simulink model "gm_sampleModel1599_2_sub"  (R2023a)
settings: Solver=VariableStepAuto  StartTime=0.0  StopTime=10.0  RelTol=1e-3
libraries: simulink x2
settings Model: Creator=user1  LastModifiedBy=user1
settings OptimizationCC: BlockReduction=off  ConditionallyExecuteInputs=off
settings DebuggingCC: InheritedTsInSrcMsg=none

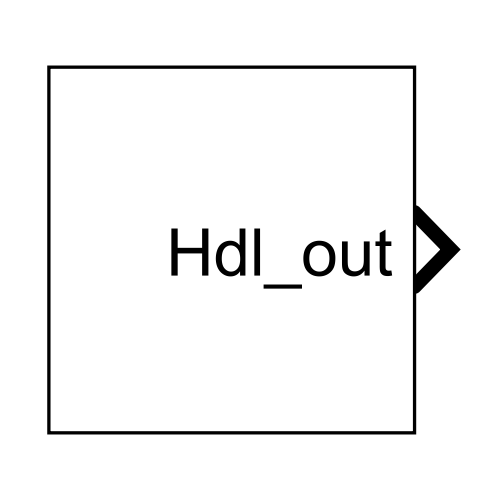
[thumbnail: Simulink's stored preview of the top-level diagram]
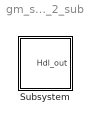
== system gm_sampleModel1599_2_sub ==
  Subsystem : Subsystem

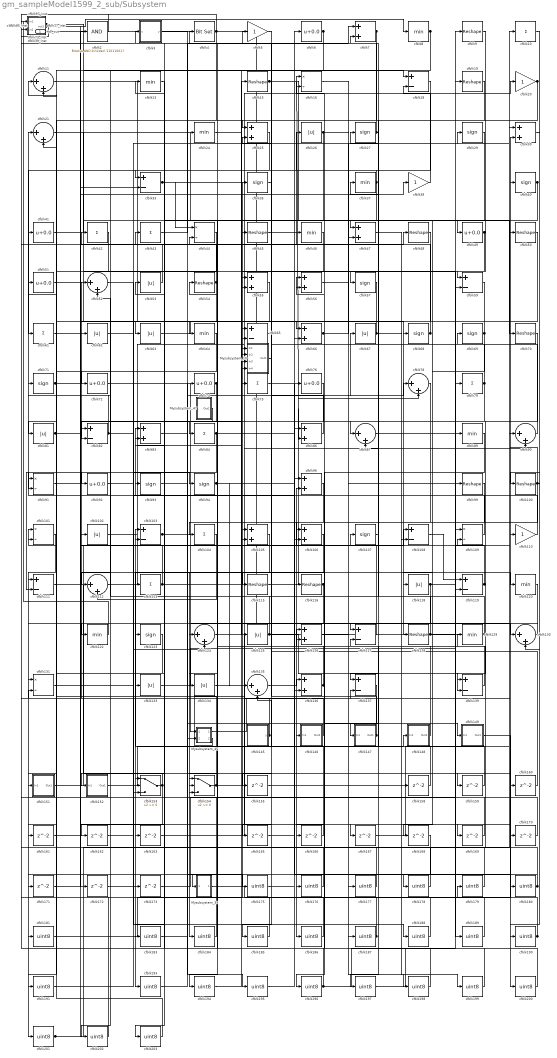
== system gm_sampleModel1599_2_sub/Subsystem ==
  Mysubsystem_10 : Subsystem
  Mysubsystem_39 : Subsystem
  Mysubsystem_45 : Subsystem
  Mysubsystem_47 : Subsystem
  cfblk1 : Constant  Value=0  OutDataTypeStr=uint8  SampleTime=1
  cfblk{10,42..43,61,75,79,84,104,113} (9 alike) : Sum  Inputs=+  OutDataTypeStr=uint8
  cfblk{9,15,19,45,48,50,54,70,99..100,115..116,128} (13 alike) : Reshape
  cfblk{16,44,91,101,109,131} (6 alike) : Product  Inputs=*/  OutDataTypeStr=uint8  RndMeth=Zero  SaturateOnIntegerOverflow=on
  cfblk{26,53,62..63,67,81,102,118,125,133..134} (11 alike) : Abs  OutDataTypeStr=uint8  SaturateOnIntegerOverflow=off
  cfblk{18,33,59,65,82,103,108,111,119,127,137,139} (12 alike) : Sum  Inputs=+-  OutDataTypeStr=uint8
  cfblk{7,25,30,47,55..56,66,83,86,96,105..106,126,136} (14 alike) : Sum  OutDataTypeStr=uint8
  cfblk{27,29,35,40,57,68..69,71,93..94,107,123} (12 alike) : Signum
  cfblk{11,21,52,78,87,90,112,124,130,135} (10 alike) : Sum  Inputs=|++  OutDataTypeStr=uint8
  cfblk{5,20,38,110} (4 alike) : Gain  OutDataTypeStr=uint8
  cfblk{8,13,24,37,46,64,89,120,122,129} (10 alike) : MinMax  OutDataTypeStr=uint8
  cfblk138_inst : Subsystem
  cfblk145 : Subsystem  mask(Counter Limited){uplimit=double(7), tsamp=double(-1)}
      mask prompts: uplimit "Simulink:masks:UpperLimit_MP"; tsamp "Simulink:masks:SampleTime_MP"
      mask help: Simulink:masks:CounterLimited_MD
      mask init:
      | nbits = double(8);
      | tsamp = double(-1);
      | uplimit = double(7);
  cfblk146 : Subsystem
  cfblk147 : Subsystem
  cfblk148 : Subsystem
  cfblk149 : Subsystem
  cfblk151 : Subsystem
  cfblk152 : Subsystem
  cfblk153 : Switch  OutDataTypeStr=uint8  SaturateOnIntegerOverflow=off  InputSameDT=off
  cfblk154 : Switch  OutDataTypeStr=uint8  SaturateOnIntegerOverflow=off  InputSameDT=off
  cfblk{155,158..163,165..173} (16 alike) : Delay  SampleTime=1
  cfblk{175..181,183..191,193..203} (27 alike) : DataTypeConversion  OutDataTypeStr=uint8  SaturateOnIntegerOverflow=off  RndMeth=Floor
  cfblk17_inst : Subsystem
  cfblk2 : simulink/Logic and Bit Operations/Bitwise Operator  logicop=AND  UseBitMask=on  BitMask=bin2dec('11011001')  BitMaskRealWorld=Stored Integer
      settings: LibrarySourceBlock=|
      | hdlsllib/Logic and Bit
      | Operations/Bitwise
      | Operator
  cfblk3 : Subsystem  mask(Compare To Zero){relop=<=, OutDataTypeStr=uint8, ZeroCross=on}
      mask prompts: relop "Simulink:masks:Operator_MP"; OutDataTypeStr "Simulink:masks:OutputDataType_MP"; ZeroCross "Simulink:masks:EnableZerocrossingDetection_MP"
      mask help: Simulink:masks:CompareToZero_MD
      mask init:
      | OutDataTypeStr = 'uint8';
      | ZeroCross = 'on';
      | blkName = 'sampleModel1599_2_sub/Subsystem/cfblk3';
      | relop = '<=';
      | setValue = 'fixdt(0, 8)';
      mask TypeOptions relop: == | ~= | < | <= | >= | >
      mask TypeOptions OutDataTypeStr: Simulink:masks:uint8 | Simulink:masks:boolean
      mask Callback ZeroCross: sl('zeroCrossEnable', gcbh);
      mask Display: disp([relop,' 0'])
  cfblk39_inst : Subsystem
  cfblk4 : simulink/Logic and Bit Operations/Bit Set  iBit=0
      settings: LibrarySourceBlock=|
      | hdlsllib/Logic and Bit
      | Operations/Bit Set
  cfblk{6,41,49,51,72,74,76,92} (8 alike) : Bias  Bias=0.0  SaturateOnIntegerOverflow=off
  cfblk73_inst : Subsystem
  cfblk77_inst : Subsystem
  cfblk85_inst : Subsystem
  cfblk97_inst : Subsystem
  Hdl_out : Outport  OutDataTypeStr=uint8  SampleTime=1
  wires:
  Mysubsystem_10/1(Out1) -> Mysubsystem_39/1(In1)
  Mysubsystem_39/1(Out1) -> cfblk30/2
  Mysubsystem_45/1(Out1) -> cfblk40/1
  Mysubsystem_45/2(Out2) -> cfblk48/1
  Mysubsystem_47/1(Out1) -> Mysubsystem_45/1(In1)
  cfblk1/1 -> cfblk87/1, cfblk63/1
  cfblk10/1 -> cfblk100/1
  cfblk100/1 -> cfblk50/1, cfblk186/1, cfblk130/2, cfblk146/1(In1)
  cfblk101/1 -> cfblk201/1
  cfblk102/1 -> cfblk20/1
  cfblk103/1 -> cfblk195/1, cfblk127/1
  cfblk104/1 -> cfblk112/2
  cfblk105/1 -> cfblk184/1
  cfblk106/1 -> cfblk193/1
  cfblk107/1 -> cfblk27/1
  cfblk108/1 -> cfblk119/1
  cfblk109/1 -> cfblk83/1
  cfblk11/1 -> cfblk128/1
  cfblk110/1 -> cfblk21/1
  cfblk111/1 -> cfblk159/1
  cfblk112/1 -> cfblk35/1
  cfblk113/1 -> cfblk52/1, cfblk15/1
  cfblk115/1 -> cfblk78/2
  cfblk116/1 -> cfblk194/1, cfblk176/1
  cfblk118/1 -> cfblk181/1, cfblk154/3, cfblk110/1
  cfblk119/1 -> cfblk52/2, cfblk109/2
  cfblk120/1 -> cfblk131/1
  cfblk122/1 -> cfblk97_inst/1(in1)
  cfblk123/1 -> cfblk151/1(In1)
  cfblk124/1 -> cfblk167/1
  cfblk125/1 -> cfblk71/1, cfblk139/2
  cfblk126/1 -> cfblk187/1
  cfblk127/1 -> cfblk96/2
  cfblk128/1 -> cfblk19/1, cfblk13/1
  cfblk129/1 -> cfblk7/2, Hdl_out/1
  cfblk13/1 -> cfblk163/1
  cfblk130/1 -> cfblk124/1
  cfblk131/1 -> cfblk173/1
  cfblk133/1 -> cfblk79/1
  cfblk134/1 -> cfblk137/2
  cfblk135/1 -> cfblk136/1
  cfblk136/1 -> cfblk85_inst/2(in2), cfblk103/1
  cfblk137/1 -> cfblk166/1
  cfblk138_inst/1(out1) -> cfblk189/1, cfblk18/1
  cfblk139/1 -> cfblk93/1
  cfblk145/1(y) -> cfblk73_inst/2(in2), cfblk62/1
  cfblk146/1(Out1) -> cfblk131/2
  cfblk147/1(Out1) -> cfblk5/1, cfblk44/2
  cfblk148/1(Out1) -> cfblk55/1
  cfblk149/1(Out1) -> cfblk200/1
  cfblk15/1 -> cfblk86/2, cfblk49/1
  cfblk151/1(Out1) -> cfblk107/1
  cfblk152/1(Out1) -> cfblk148/1(In1)
  cfblk153/1 -> cfblk162/1, cfblk152/1(In1)
  cfblk154/1 -> cfblk90/2, cfblk21/2
  cfblk155/1 -> cfblk66/2
  cfblk158/1 -> cfblk127/2
  cfblk159/1 -> cfblk103/2
  cfblk16/1 -> cfblk177/1
  cfblk160/1 -> cfblk25/2
  cfblk161/1 -> cfblk108/1
  cfblk162/1 -> cfblk188/1
  cfblk163/1 -> cfblk78/1
  cfblk165/1 -> cfblk136/2
  cfblk166/1 -> cfblk135/2
  cfblk167/1 -> cfblk90/1
  cfblk168/1 -> cfblk178/1
  cfblk169/1 -> cfblk17_inst/1(in1)
  cfblk17_inst/1(out1) -> cfblk57/1
  cfblk170/1 -> cfblk83/2
  cfblk171/1 -> cfblk59/2
  cfblk172/1 -> cfblk96/1
  cfblk173/1 -> cfblk109/1
  cfblk175/1 -> cfblk76/1
  cfblk176/1 -> cfblk3/1(u)
  cfblk177/1 -> cfblk17_inst/2(in2)
  cfblk178/1 -> cfblk16/1
  cfblk179/1 -> cfblk16/2
  cfblk18/1 -> cfblk82/2
  cfblk180/1 -> cfblk4/1, cfblk171/1, cfblk129/1
  cfblk181/1 -> cfblk75/1
  cfblk183/1 -> Mysubsystem_45/2(In2)
  cfblk184/1 -> cfblk53/1
  cfblk185/1 -> cfblk105/1
  cfblk186/1 -> cfblk105/2
  cfblk187/1 -> cfblk86/1, cfblk77_inst/2(in2)
  cfblk188/1 -> cfblk126/1
  cfblk189/1 -> cfblk126/2
  cfblk19/1 -> cfblk47/1
  cfblk190/1 -> cfblk179/1, cfblk138_inst/1(in1)
  cfblk191/1 -> cfblk30/1
  cfblk193/1 -> cfblk67/1
  cfblk194/1 -> cfblk106/1
  cfblk195/1 -> cfblk106/2
  cfblk196/1 -> cfblk97_inst/2(in2), cfblk9/1, cfblk43/1
  cfblk197/1 -> cfblk89/1
  cfblk198/1 -> cfblk54/1
  cfblk199/1 -> cfblk56/1
  cfblk2/1 -> cfblk39_inst/1(in1)
  cfblk20/1 -> cfblk81/1, cfblk203/1
  cfblk200/1 -> cfblk56/2
  cfblk201/1 -> cfblk2/1, cfblk10/1
  cfblk202/1 -> cfblk101/1
  cfblk203/1 -> cfblk101/2
  cfblk21/1 -> cfblk70/1
  cfblk24/1 -> cfblk65/1
  cfblk25/1 -> cfblk61/1
  cfblk26/1 -> cfblk99/1, cfblk165/1
  cfblk27/1 -> cfblk87/2, cfblk85_inst/1(in1), cfblk197/1
  cfblk29/1 -> cfblk147/1(In1)
  cfblk3/1(y) -> cfblk175/1
  cfblk30/1 -> cfblk190/1
  cfblk33/1 -> cfblk116/1, cfblk44/1, Mysubsystem_10/3(In3)
  cfblk35/1 -> cfblk115/1
  cfblk37/1 -> cfblk33/1, cfblk134/1
  cfblk38/1 -> cfblk18/2
  cfblk39_inst/1(out1) -> cfblk8/1
  cfblk4/1 -> cfblk73_inst/1(in1), cfblk153/1
  cfblk40/1 -> cfblk47/2, cfblk183/1
  cfblk41/1 -> cfblk24/1
  cfblk42/1 -> cfblk161/1
  cfblk43/1 -> cfblk7/1
  cfblk44/1 -> cfblk91/2
  cfblk45/1 -> cfblk26/1
  cfblk46/1 -> cfblk185/1
  cfblk47/1 -> cfblk199/1
  cfblk48/1 -> cfblk112/1
  cfblk49/1 -> cfblk55/2, Mysubsystem_10/4(In4)
  cfblk5/1 -> cfblk25/1
  cfblk50/1 -> cfblk153/3
  cfblk51/1 -> cfblk84/1
  cfblk52/1 -> cfblk124/2
  cfblk53/1 -> cfblk77_inst/1(in1)
  cfblk54/1 -> cfblk153/2, cfblk42/1
  cfblk55/1 -> cfblk91/1
  cfblk56/1 -> cfblk198/1
  cfblk57/1 -> cfblk92/1
  cfblk59/1 -> cfblk118/1
  cfblk6/1 -> Mysubsystem_10/1(In1), cfblk122/1
  cfblk61/1 -> cfblk102/1
  cfblk62/1 -> cfblk154/2
  cfblk63/1 -> cfblk66/1
  cfblk64/1 -> cfblk111/1
  cfblk65/1 -> cfblk113/1
  cfblk66/1 -> cfblk68/1, cfblk29/1, cfblk130/1
  cfblk67/1 -> cfblk72/1, cfblk169/1
  cfblk68/1 -> cfblk11/1, cfblk37/1
  cfblk69/1 -> cfblk65/2, cfblk168/1
  cfblk7/1 -> cfblk155/1, Mysubsystem_10/2(In2)
  cfblk70/1 -> cfblk139/1
  cfblk71/1 -> cfblk170/1, cfblk46/1
  cfblk72/1 -> cfblk125/1
  cfblk73_inst/1(out1) -> cfblk33/2, cfblk64/1
  cfblk74/1 -> cfblk202/1, cfblk123/1
  cfblk75/1 -> cfblk180/1
  cfblk76/1 -> cfblk133/1
  cfblk77_inst/1(out1) -> cfblk39_inst/2(in2)
  cfblk78/1 -> cfblk108/2
  cfblk79/1 -> cfblk69/1, cfblk154/1
  cfblk8/1 -> cfblk82/1, cfblk11/2
  cfblk81/1 -> cfblk191/1, cfblk119/2
  cfblk82/1 -> cfblk51/1, cfblk160/1
  cfblk83/1 -> cfblk74/1
  cfblk84/1 -> cfblk111/2, cfblk158/1
  cfblk85_inst/1(out1) -> cfblk172/1
  cfblk86/1 -> cfblk45/1
  cfblk87/1 -> cfblk120/1
  cfblk89/1 -> cfblk196/1
  cfblk9/1 -> cfblk59/1
  cfblk90/1 -> cfblk41/1
  cfblk91/1 -> cfblk38/1
  cfblk92/1 -> cfblk94/1
  cfblk93/1 -> cfblk149/1(In1)
  cfblk94/1 -> cfblk6/1, cfblk135/1
  cfblk96/1 -> cfblk104/1
  cfblk97_inst/1(out1) -> cfblk138_inst/2(in2)
  cfblk99/1 -> cfblk137/1

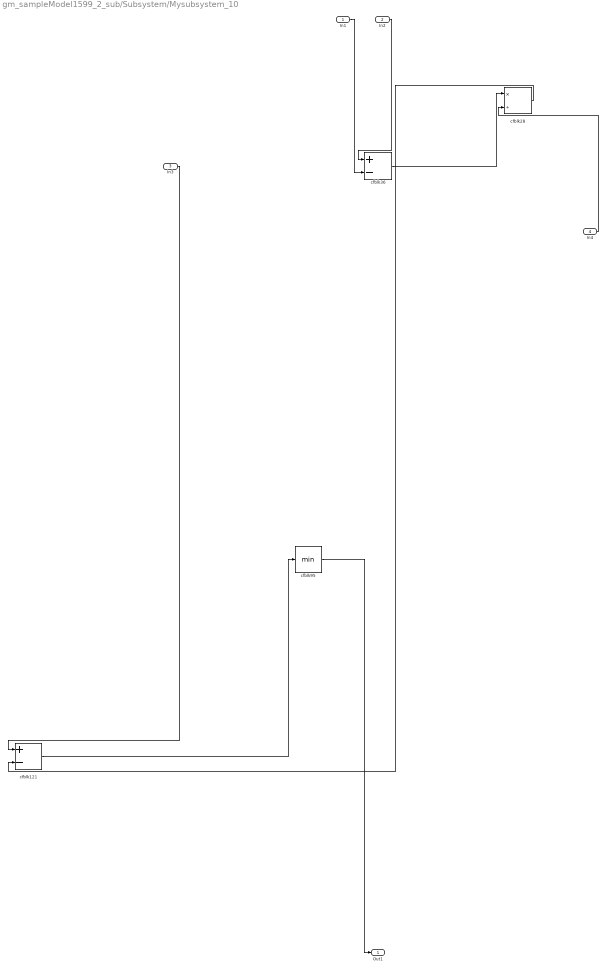
== system gm_sampleModel1599_2_sub/Subsystem/Mysubsystem_10 ==
  In1 : Inport  OutDataTypeStr=uint8  PortDimensions=1  SampleTime=1
  In2 : Inport  Port=2  OutDataTypeStr=uint8  PortDimensions=1  SampleTime=1
  In3 : Inport  Port=3  OutDataTypeStr=uint8  PortDimensions=1  SampleTime=1
  In4 : Inport  Port=4  OutDataTypeStr=uint8  PortDimensions=1  SampleTime=1
  cfblk121 : Sum  Inputs=+-
  cfblk28 : Product  Inputs=*/  RndMeth=Zero  SaturateOnIntegerOverflow=on
  cfblk36 : Sum  Inputs=+-
  cfblk95 : MinMax
  Out1 : Outport  SampleTime=1
  wires:
  In1/1 -> cfblk36/2
  In2/1 -> cfblk36/1
  In3/1 -> cfblk121/1
  In4/1 -> cfblk28/2
  cfblk121/1 -> cfblk95/1
  cfblk28/1 -> cfblk121/2
  cfblk36/1 -> cfblk28/1
  cfblk95/1 -> Out1/1

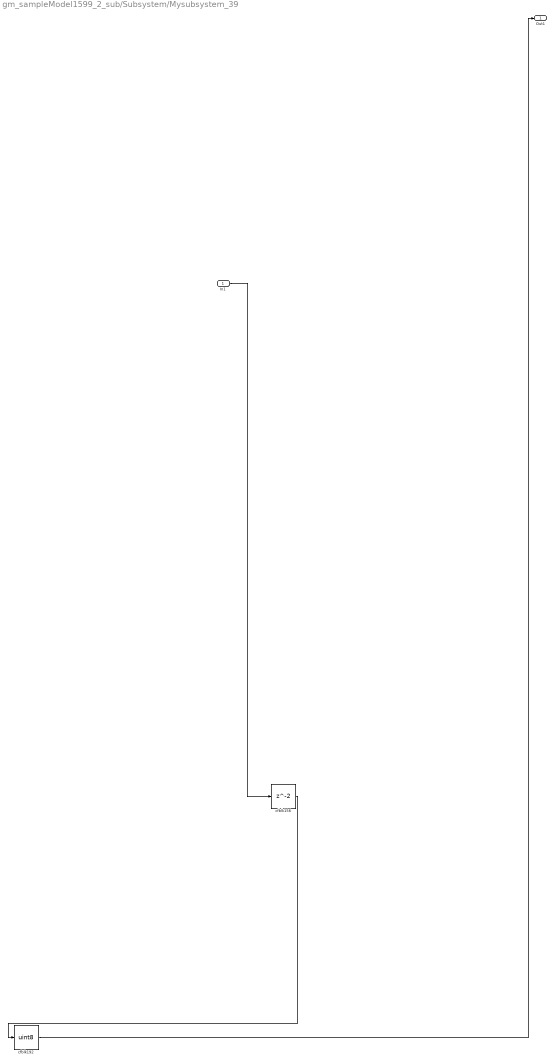
== system gm_sampleModel1599_2_sub/Subsystem/Mysubsystem_39 ==
  In1 : Inport  OutDataTypeStr=uint8  PortDimensions=1  SampleTime=1
  cfblk156 : Delay  SampleTime=1
  cfblk192 : DataTypeConversion  OutDataTypeStr=uint8  SaturateOnIntegerOverflow=off  RndMeth=Floor
  Out1 : Outport  SampleTime=1
  wires:
  In1/1 -> cfblk156/1
  cfblk156/1 -> cfblk192/1
  cfblk192/1 -> Out1/1

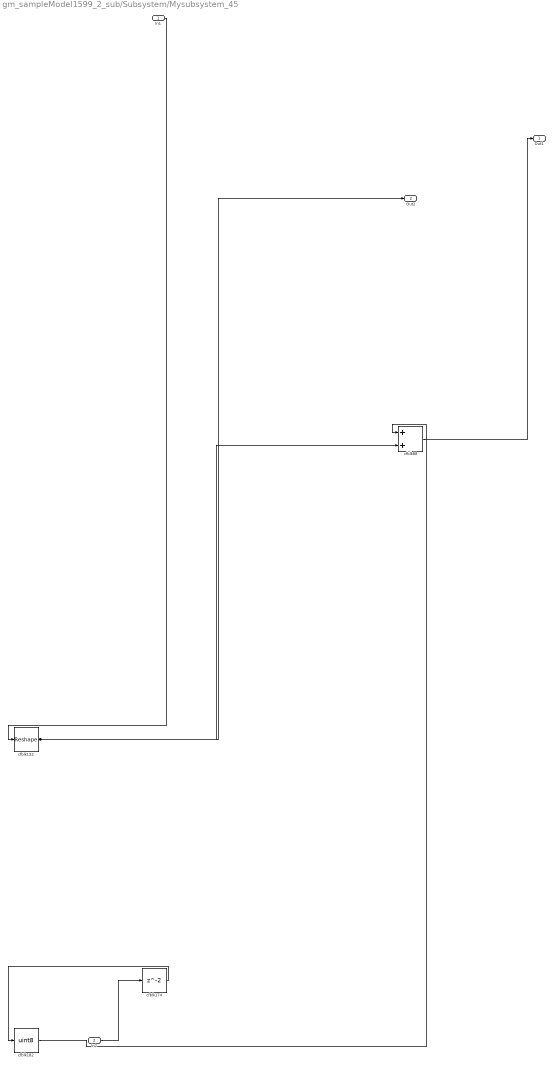
== system gm_sampleModel1599_2_sub/Subsystem/Mysubsystem_45 ==
  In1 : Inport  OutDataTypeStr=uint8  PortDimensions=1  SampleTime=1
  In2 : Inport  Port=2  OutDataTypeStr=uint8  PortDimensions=1  SampleTime=1
  cfblk132 : Reshape
  cfblk174 : Delay  SampleTime=1
  cfblk182 : DataTypeConversion  OutDataTypeStr=uint8  SaturateOnIntegerOverflow=off  RndMeth=Floor
  cfblk88 : Sum
  Out1 : Outport  SampleTime=1
  Out2 : Outport  Port=2  SampleTime=1
  wires:
  In1/1 -> cfblk132/1
  In2/1 -> cfblk174/1
  cfblk132/1 -> cfblk88/2, Out2/1
  cfblk174/1 -> cfblk182/1
  cfblk182/1 -> cfblk88/1
  cfblk88/1 -> Out1/1

== system gm_sampleModel1599_2_sub/Subsystem/Mysubsystem_47 ==
  cfblk14 : Reshape
  cfblk144 : Ground
  Out1 : Outport  SampleTime=1
  wires:
  cfblk14/1 -> Out1/1
  cfblk144/1 -> cfblk14/1

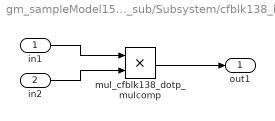
== system gm_sampleModel1599_2_sub/Subsystem/cfblk138_inst ==
  in1 : Inport  OutDataTypeStr=uint8  SampleTime=1
  in2 : Inport  Port=2  OutDataTypeStr=uint8  SampleTime=1
  mul_cfblk138_dotp_mulcomp : Product  Inputs=**  OutDataTypeStr=uint8  SampleTime=1
  out1 : Outport  OutDataTypeStr=uint8  SampleTime=1
  wires:
  in1/1 -> mul_cfblk138_dotp_mulcomp/1
  in2/1 -> mul_cfblk138_dotp_mulcomp/2
  mul_cfblk138_dotp_mulcomp/1 -> out1/1

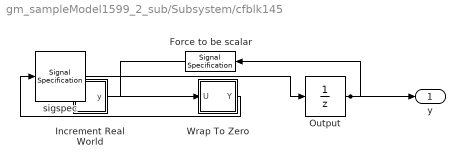
== system gm_sampleModel1599_2_sub/Subsystem/cfblk145 ==
  Force to be scalar : SignalSpecification  DisableCoverage=on  Dimensions=1
  Increment Real World : Subsystem  mask(Real World Value Increment){}
      mask help: Simulink:masks:RealWorldValueIncrement_MD
      mask Display: disp('V++')
  Output : UnitDelay  InitialCondition=0.0  SampleTime=tsamp  HasFrameUpgradeWarning=on
  Wrap To Zero : Subsystem  mask(Wrap To Zero){Threshold=double(7)}
      mask prompts: Threshold "Simulink:masks:Threshold_MP"
      mask help: Simulink:masks:WrapToZero_MD
  sigspec : SignalSpecification  OutDataTypeStr=uint8  Dimensions=1
  y : Outport  SampleTime=1
  wires:
  Force to be scalar/1 -> Increment Real World/1(u)
  Increment Real World/1(y) -> Wrap To Zero/1(U)
  Output/1 -> Force to be scalar/1, y/1
  Wrap To Zero/1(Y) -> sigspec/1
  sigspec/1 -> Output/1

== system gm_sampleModel1599_2_sub/Subsystem/cfblk146 ==
  In1 : Inport  OutDataTypeStr=uint8  PortDimensions=1  SampleTime=1
  Out1 : Outport  SampleTime=1
  wires:
  In1/1 -> Out1/1

== system gm_sampleModel1599_2_sub/Subsystem/cfblk147 ==
  In1 : Inport  OutDataTypeStr=uint8  PortDimensions=1  SampleTime=1
  Out1 : Outport  SampleTime=1
  wires:
  In1/1 -> Out1/1

== system gm_sampleModel1599_2_sub/Subsystem/cfblk148 ==
  In1 : Inport  OutDataTypeStr=uint8  PortDimensions=1  SampleTime=1
  Out1 : Outport  SampleTime=1
  wires:
  In1/1 -> Out1/1

== system gm_sampleModel1599_2_sub/Subsystem/cfblk149 ==
  In1 : Inport  OutDataTypeStr=uint8  PortDimensions=1  SampleTime=1
  Out1 : Outport  SampleTime=1
  wires:
  In1/1 -> Out1/1

== system gm_sampleModel1599_2_sub/Subsystem/cfblk151 ==
  In1 : Inport  OutDataTypeStr=uint8  PortDimensions=1  SampleTime=1
  Out1 : Outport  SampleTime=1
  wires:
  In1/1 -> Out1/1

== system gm_sampleModel1599_2_sub/Subsystem/cfblk152 ==
  In1 : Inport  OutDataTypeStr=uint8  PortDimensions=1  SampleTime=1
  Out1 : Outport  SampleTime=1
  wires:
  In1/1 -> Out1/1

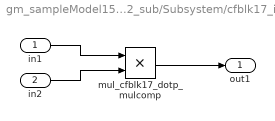
== system gm_sampleModel1599_2_sub/Subsystem/cfblk17_inst ==
  in1 : Inport  OutDataTypeStr=uint8  SampleTime=1
  in2 : Inport  Port=2  OutDataTypeStr=uint8  SampleTime=1
  mul_cfblk17_dotp_mulcomp : Product  Inputs=**  OutDataTypeStr=uint8  SampleTime=1
  out1 : Outport  OutDataTypeStr=uint8  SampleTime=1
  wires:
  in1/1 -> mul_cfblk17_dotp_mulcomp/1
  in2/1 -> mul_cfblk17_dotp_mulcomp/2
  mul_cfblk17_dotp_mulcomp/1 -> out1/1

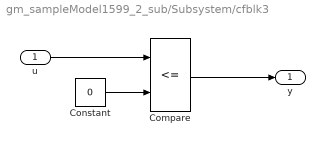
== system gm_sampleModel1599_2_sub/Subsystem/cfblk3 ==
  u : Inport  OutDataTypeStr=uint8  SampleTime=1
  Compare : RelationalOperator  Operator=<=  OutDataTypeStr=fixdt(0, 8)
  Constant : Constant  DisableCoverage=on  Value=0  OutDataTypeStr=Inherit: Inherit via back propagation  SampleTime=-1  PreserveConstantTs=on
  y : Outport  SampleTime=1
  wires:
  u/1 -> Compare/1
  Compare/1 -> y/1
  Constant/1 -> Compare/2

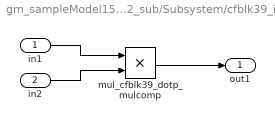
== system gm_sampleModel1599_2_sub/Subsystem/cfblk39_inst ==
  in1 : Inport  OutDataTypeStr=uint8  SampleTime=1
  in2 : Inport  Port=2  OutDataTypeStr=uint8  SampleTime=1
  mul_cfblk39_dotp_mulcomp : Product  Inputs=**  OutDataTypeStr=uint8  SampleTime=1
  out1 : Outport  OutDataTypeStr=uint8  SampleTime=1
  wires:
  in1/1 -> mul_cfblk39_dotp_mulcomp/1
  in2/1 -> mul_cfblk39_dotp_mulcomp/2
  mul_cfblk39_dotp_mulcomp/1 -> out1/1

== system gm_sampleModel1599_2_sub/Subsystem/cfblk73_inst ==
  in1 : Inport  OutDataTypeStr=uint8  SampleTime=1
  in2 : Inport  Port=2  OutDataTypeStr=uint8  SampleTime=1
  mul_cfblk73_dotp_mulcomp : Product  Inputs=**  OutDataTypeStr=uint8  SampleTime=1
  out1 : Outport  OutDataTypeStr=uint8  SampleTime=1
  wires:
  in1/1 -> mul_cfblk73_dotp_mulcomp/1
  in2/1 -> mul_cfblk73_dotp_mulcomp/2
  mul_cfblk73_dotp_mulcomp/1 -> out1/1

== system gm_sampleModel1599_2_sub/Subsystem/cfblk77_inst ==
  in1 : Inport  OutDataTypeStr=uint8  SampleTime=1
  in2 : Inport  Port=2  OutDataTypeStr=uint8  SampleTime=1
  mul_cfblk77_dotp_mulcomp : Product  Inputs=**  OutDataTypeStr=uint8  SampleTime=1
  out1 : Outport  OutDataTypeStr=uint8  SampleTime=1
  wires:
  in1/1 -> mul_cfblk77_dotp_mulcomp/1
  in2/1 -> mul_cfblk77_dotp_mulcomp/2
  mul_cfblk77_dotp_mulcomp/1 -> out1/1

== system gm_sampleModel1599_2_sub/Subsystem/cfblk85_inst ==
  in1 : Inport  OutDataTypeStr=uint8  SampleTime=1
  in2 : Inport  Port=2  OutDataTypeStr=uint8  SampleTime=1
  mul_cfblk85_dotp_mulcomp : Product  Inputs=**  OutDataTypeStr=uint8  SampleTime=1
  out1 : Outport  OutDataTypeStr=uint8  SampleTime=1
  wires:
  in1/1 -> mul_cfblk85_dotp_mulcomp/1
  in2/1 -> mul_cfblk85_dotp_mulcomp/2
  mul_cfblk85_dotp_mulcomp/1 -> out1/1

== system gm_sampleModel1599_2_sub/Subsystem/cfblk97_inst ==
  in1 : Inport  OutDataTypeStr=uint8  SampleTime=1
  in2 : Inport  Port=2  OutDataTypeStr=uint8  SampleTime=1
  mul_cfblk97_dotp_mulcomp : Product  Inputs=**  OutDataTypeStr=uint8  SampleTime=1
  out1 : Outport  OutDataTypeStr=uint8  SampleTime=1
  wires:
  in1/1 -> mul_cfblk97_dotp_mulcomp/1
  in2/1 -> mul_cfblk97_dotp_mulcomp/2
  mul_cfblk97_dotp_mulcomp/1 -> out1/1

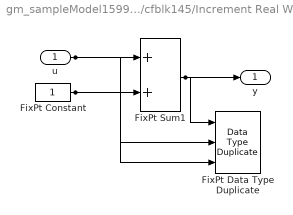
== system gm_sampleModel1599_2_sub/Subsystem/cfblk145/Increment Real World ==
  u : Inport  OutDataTypeStr=uint8  SampleTime=1
  FixPt Constant : Constant  DisableCoverage=on  OutDataTypeStr=Inherit: Inherit via back propagation  SampleTime=-1
  FixPt Data Type Duplicate : DataTypeDuplicate  DisableCoverage=on  NumInputPorts=3
  FixPt Sum1 : Sum  InputSameDT=on  OutDataTypeStr=Inherit: Inherit via back propagation  LockScale=on
  y : Outport  SampleTime=1
  wires:
  u/1 -> FixPt Sum1/1, FixPt Data Type Duplicate/2
  FixPt Constant/1 -> FixPt Sum1/2, FixPt Data Type Duplicate/3
  FixPt Sum1/1 -> FixPt Data Type Duplicate/1, y/1

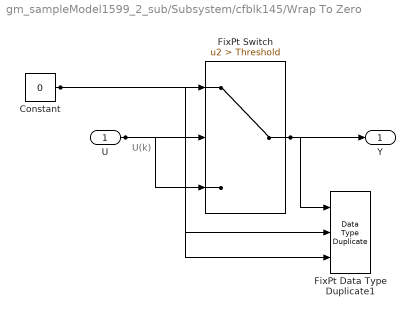
== system gm_sampleModel1599_2_sub/Subsystem/cfblk145/Wrap To Zero ==
  note: U(k)
  U : Inport  OutDataTypeStr=uint8  SampleTime=1
  Constant : Constant  DisableCoverage=on  Value=0  OutDataTypeStr=Inherit: Inherit via back propagation  SampleTime=-1
  FixPt Data Type Duplicate1 : DataTypeDuplicate  DisableCoverage=on  NumInputPorts=3
  FixPt Switch : Switch  Criteria=u2 > Threshold  Threshold=Threshold  OutDataTypeStr=Inherit: Inherit via back propagation  ZeroCross=off  SaturateOnIntegerOverflow=off  InputSameDT=off
  Y : Outport  SampleTime=1
  wires:
  U/1 -> FixPt Switch/3, FixPt Switch/2, FixPt Data Type Duplicate1/2
  Constant/1 -> FixPt Switch/1, FixPt Data Type Duplicate1/3
  FixPt Switch/1 -> FixPt Data Type Duplicate1/1, Y/1
